simulink model "SimulacaoMotorCCr2015a"  (R2015a)
settings: Solver=ode3  SolverMode=SingleTasking  StartTime=0.0  StopTime=0.23  RelTol=1e-4
values from neighbouring files (symbols this model uses):
  B = 1.8e-3    (= 0.0018)    [ParameterEstimation.m]    (also in ParameterEstimation_moodle.m = 0.0006)
  J = 1.1e-5    (= 1.1e-05)    [ParameterEstimation.m]    (also in ParameterEstimation_moodle.m = 0.00050804)
  K = 0.0673    [ParameterEstimation.m]    (also in ParameterEstimation_moodle.m = 0.087)
  La = 0.5e-3    (= 0.0005)    [ParameterEstimation.m]    (also in ParameterEstimation_moodle.m = 0.00015)
  Ra = 2.47    [ParameterEstimation.m]    (also in ParameterEstimation_moodle.m = 0.1501)
  Ts = 4e-4    (= 0.0004)    [ParameterEstimation.m]    (also in ParameterEstimation_moodle.m = 0.0001)
Description:
  | Sistema de injeção completo.
settings Model: CovModelRefEnable=off  ExtModeAutoUpdateStatusClock=off  Creator=vtchkalo  LastModifiedBy=Lucas Jonys
settings SolverCC: MaxConsecutiveZCs=100000  ZeroCrossAlgorithm=Adaptive
settings DataIOCC: SaveState=on  SignalLogging=off  DSMLogging=off  OutputOption=SpecifiedOutputTimes  OutputTimes=SDO_OutputTimes  ReturnWorkspaceOutputsName=SDOSimTest_Log
settings OptimizationCC: BlockReduction=off  BooleanDataType=off
settings DebuggingCC: SaveWithParameterizedLinksMsg=none  UnderspecifiedInitializationDetection=Classic  MergeDetectMultiDrivingBlocksExec=none  SignalResolutionControl=TryResolveAllWithWarning  MultiTaskDSMMsg=warning  MultiTaskCondExecSysMsg=none  StateNameClashWarn=warning
settings HardwareCC: TargetUnknown=on
settings GRTTargetCC: GeneratePreprocessorConditionals=Use local settings
settings ConfigurationSet: Description=Simscape Multibody

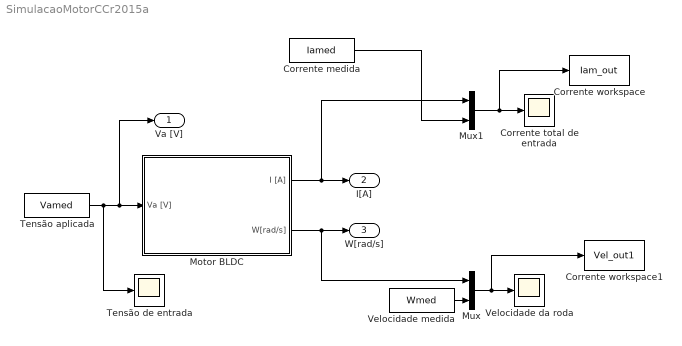
== system SimulacaoMotorCCr2015a ==
  Corrente medida : FromWorkspace  VariableName=Iamed  SampleTime=Ts
  Corrente total de entrada : Scope
      settings: TimeRange=auto  MaxDataPoints=5000  SaveToWorkspace=off  YMin=-8.54468  YMax=76.90208  SampleTime=-1
  Corrente workspace : ToWorkspace  VariableName=Iam_out  SaveFormat=Timeseries  SampleTime=-1
  Corrente workspace1 : ToWorkspace  VariableName=Vel_out1  SaveFormat=Timeseries  SampleTime=-1
  Motor BLDC : Subsystem
  Mux : Mux  Inputs=2
  Mux1 : Mux  Inputs=2
  Tensão aplicada : FromWorkspace  VariableName=Vamed  SampleTime=Ts
  Tensão de entrada : Scope
      settings: TimeRange=auto  MaxDataPoints=5000  SaveToWorkspace=off  YMin=2.28  YMax=22.28  SampleTime=-1
  Velocidade da roda : Scope
      settings: TimeRange=auto  MaxDataPoints=5000  SaveName=ScopeData  YMin=-20.94415  YMax=188.49734  SampleTime=-1
  Velocidade medida : FromWorkspace  VariableName=Wmed  SampleTime=Ts
  Va [V] : Outport
  I[A] : Outport  Port=2
  W[rad/s] : Outport  Port=3
  wires:
  Tensão aplicada/1 -> Motor BLDC/1(Va [V]), Va [V]/1, Tensão de entrada/1
  Velocidade medida/1 -> Mux/2
  Mux/1 -> Corrente workspace1/1, Velocidade da roda/1
  Mux1/1 -> Corrente workspace/1, Corrente total de entrada/1
  Corrente medida/1 -> Mux1/2
  Motor BLDC/1(I [A]) -> Mux1/1, I[A]/1
  Motor BLDC/2(W[rad/s]) -> Mux/1, W[rad/s]/1

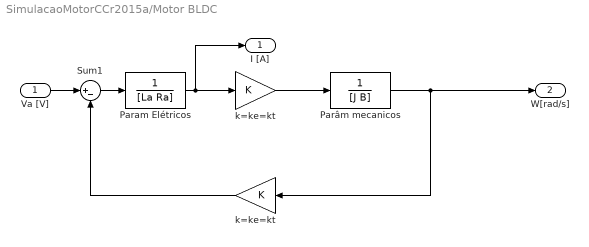
== system SimulacaoMotorCCr2015a/Motor BLDC ==
  Va [V] : Inport
  Param Elétricos : TransferFcn  Denominator=[La Ra]
  Parâm mecanicos : TransferFcn  Denominator=[J B]
  Sum1 : Sum  Inputs=|+-
  k=ke=kt : Gain  Gain=K
  "k=ke=kt " : Gain  Gain=K
  I [A] : Outport
  W[rad/s] : Outport  Port=2
  wires:
  Sum1/1 -> Param Elétricos/1
  Va [V]/1 -> Sum1/1
  k=ke=kt/1 -> Sum1/2
  "k=ke=kt "/1 -> Parâm mecanicos/1
  Param Elétricos/1 -> I [A]/1, "k=ke=kt "/1
  Parâm mecanicos/1 -> W[rad/s]/1, k=ke=kt/1
